simulink model "rev0BB"  (R2017b)
settings: Solver=FixedStepDiscrete  StartTime=0  StopTime=(((preLen+100+dataLenSymbols)*1+pad_first*3)*basePer)  RelTol=1e-3
values from neighbouring files (symbols this model uses):
  ack_stf_len_symbols = length(x_ACK_STF)    [rev0BB_setup.m]
  agc_delay_lag = 32    [rev0BB_setup.m]
  agc_detector_coef = ones(1,agc_detector_taps)./agc_detector_taps    [rev0BB_setup.m]
  agc_on = true    [rev0BB_startup.m]
  agc_sat_low = -agcSaturation    (= -12)    [rev0BB_setup.m]
  agc_sat_up = agcSaturation    (= 12)    [rev0BB_setup.m]
  agcDesired = 0    [rev0BB_setup.m]
  agcExpDomain = agcSaturation    (= 12)    [rev0BB_setup.m]
  agcExpResolution = 2^-5    (= 0.03125)    [rev0BB_setup.m]
  agcPwrAvgNum = 128    [rev0BB_setup.m]
  agcSaturation = 12    [rev0BB_setup.m]
  agcSettleThresh = 0.65    [rev0BB_setup.m]
  agcStep = 2^-8    (= 0.00390625)    [rev0BB_setup.m]
  atanDomain = 5    [rev0BB_setup.m]
  atanDomainTiming = 256    [rev0BB_setup.m]
  atanResolution = 2^-9    (= 0.001953125)    [rev0BB_setup.m]
  atanResolutionTiming = 2^-5    (= 0.03125)    [rev0BB_setup.m]
  averaging_num = ones(1, averaging_samples)    [rev0BB_setup.m]
  averaging_samples = 128    [rev0BB_setup.m]
  awgnSeed = abs(dBSnrRange(dBSnrInd)*1000+trial+10000000)    [plotBer.m]    (also in rev0BB_startup.m = 67)
  basePer = 1/baseFreq    (= 5e-08)    [rev0BB_setup.m]
  bitsPerSymbolHeader = log2(radixHeader)    [rev0BB_setup.m]
  bitsPerSymbolMax = log2(radixMax)    [rev0BB_setup.m]
  cal_sig_i_mult = 1.0    (= 1)    [rev0BB_startup.m]
  cal_sig_i_offset = 0.0    (= 0)    [rev0BB_startup.m]
  cal_sig_q_mult = 1.0    (= 1)    [rev0BB_startup.m]
  cal_sig_q_offset = 0.0    (= 0)    [rev0BB_startup.m]
  cefEarlyWarning = 256    [rev0BB_setup.m]
  cefLen = length(x_CEF)    [rev0BB_setup.m]
  channelFIR = zeros(1, round(maxSampleDelay)+1)    [rev0BB_startup.m]
  coarseCFOAdaptDelay = 1    [rev0BB_setup.m]
  cr_i = 0.020    (= 0.02)    [rev0BB_setup.m]
  cr_i_preamp = 2^-9    (= 0.001953125)    [rev0BB_setup.m]
  cr_int1_sat_low = -cr_integrator1_saturation    (= -0.6)    [rev0BB_setup.m]
  cr_int1_sat_up = cr_integrator1_saturation    (= 0.6)    [rev0BB_setup.m]
  cr_integrator1_decay = 1    [rev0BB_setup.m]
  cr_integrator1_saturation = 0.6    [rev0BB_setup.m]
  cr_mult_pipeline = 0    [rev0BB_setup.m]
  cr_p = 0.015    [rev0BB_setup.m]
  cr_sat2_low = -cr_saturation2    (= -0.6)    [rev0BB_setup.m]
  cr_sat2_up = cr_saturation2    (= 0.6)    [rev0BB_setup.m]
  cr_smooth_num = (1/cr_smooth_samples).*ones(1, cr_smooth_samples)    [rev0BB_setup.m]
  D_128 = [ 1,  8,  2,  4, 16, 32, 64]    [golay.m]    (also in rev0BB_setup.m)
  D_32 = [ 1,  4,  8,  2, 16]    [golay.m]    (also in rev0BB_setup.m)
  dataLenSymbols = header_len_bytes*8/bitsPerSymbolHeader + frame_len_bytes*8/bitsPerSymbol    [rev0BB_setup.m]
  default_channel = 3    [rev0BB_setup.m]
  dmm_coefs = ones(1,dmm_samples)./dmm_samples    [rev0BB_setup.m]
  dst_field_len = 8    [rev0BB_setup.m]
  expDomain = 3.3    [rev0BB_setup.m]
  expResolution = 2^-5    (= 0.03125)    [rev0BB_setup.m]
  expTol = .1    (= 0.1)    [rev0BB_setup.m]
  flush_delay = regular_pipeline*2+mult_pipeline+4    (= 4)    [rev0BB_setup.m]
  frac_lut_domain = 256    [rev0BB_setup.m]
  frac_lut_domain_cr = 64    [rev0BB_setup.m]
  frac_lut_range_max = 512    [rev0BB_setup.m]
  frac_lut_range_max_coarse_cfo = 127    [rev0BB_setup.m]
  frac_lut_range_max_cr = 127    [rev0BB_setup.m]
  frac_lut_range_min = -frac_lut_range_max    (= -512)    [rev0BB_setup.m]
  frac_lut_range_min_coarse_cfo = -frac_lut_range_max_coarse_cfo    (= -127)    [rev0BB_setup.m]
  frac_lut_range_min_cr = -frac_lut_range_max_cr    (= -127)    [rev0BB_setup.m]
  frac_lut_table_breaks = -frac_lut_domain:frac_lut_res:(frac_lut_domain-1)    [rev0BB_setup.m]
  frac_lut_table_breaks_coarse_cfo = -frac_lut_domain_coarse_cfo:frac_lut_res_coarse_cfo:(frac_lut_domain_coarse_cfo-1)    [rev0BB_setup.m]
  frac_lut_table_breaks_cr = -frac_lut_domain_cr:frac_lut_res_cr:(frac_lut_domain_cr-1)    [rev0BB_setup.m]
  frac_lut_table_data = 1./frac_lut_table_breaks    [rev0BB_setup.m]
  frac_lut_table_data_coarse_cfo = 1./frac_lut_table_breaks_coarse_cfo    [rev0BB_setup.m]
  frac_lut_table_data_cr = 1./frac_lut_table_breaks_cr    [rev0BB_setup.m]
  freeze_en_agc = true    [rev0BB_startup.m]
  freeze_en_cr_int1 = false    [rev0BB_startup.m]
  freeze_en_cr_int2 = false    [rev0BB_startup.m]
  freeze_en_cr_phase = false    [rev0BB_startup.m]
  freeze_en_tr_int1 = false    [rev0BB_startup.m]
  freeze_en_tr_int2 = false    [rev0BB_startup.m]
  freeze_en_tr_phase = false    [rev0BB_startup.m]
  freeze_on_cef_done = true    [rev0BB_startup.m]
  freeze_on_stf_done = false    [rev0BB_startup.m]
  freeze_on_valid = true    [rev0BB_startup.m]
  golay_type = 32    [rev0BB_setup.m]
  guardInt = int16(4)    [rev0BB_setup.m]
  guardTol = int16(5)    [rev0BB_setup.m]
  header_len_bytes = 8    [rev0BB_setup.m]
  lineWidth = 60    [rev0BB_setup.m]
  lmsEqDepth = 38    [rev0BB_setup.m]
  lmsStep_init = 0.006    [rev0BB_setup.m]
  lmsStep_meta = (lmsStep_final - lmsStep_init)/cefLen    [rev0BB_setup.m]
  lnDomain = 16    [rev0BB_setup.m]
  lnResolution = 2^-5    (= 0.03125)    [rev0BB_setup.m]
  local_node_id = 2    [rev0BB_startup.m]
  maxMsgSize = length(xSpectrum_PRE)+dataLenSymbols+300    [rev0BB_setup.m]
  minSTFPeaks = 3    [rev0BB_setup.m]
  mod_scheme_len_bytes = 1    [rev0BB_setup.m]
  modBPS = [1, 2, 4]    [rev0BB_setup.m]
  modKeys = [0, 1, 2]    [rev0BB_setup.m]
  mult_pipeline = 0    [rev0BB_setup.m]
  overSampleFreq = 80e6    (= 80000000)    [rev0BB_setup.m]
  overSamplePer = 1/overSampleFreq    (= 1.25e-08)    [rev0BB_setup.m]
  pad_first = 1000    [createTestVectors.m]
  post_cr_i_offset = 0    [rev0BB_startup.m]
  post_cr_q_offset = 0    [rev0BB_startup.m]
  preambleSequentialDetect = 2    [rev0BB_setup.m]
  preLen = length(x_PRE)    [rev0BB_setup.m]
  qam16_demod_scale_factor = qam16_hdl_distance/qam16_power_normalized_distance    [rev0BB_setup.m]
  rcRxFilt = [0.000303163120401141 -0.00118915940834234 -0.00187387637177 -0.00124167532697737 0.00029186889076529 0.00164526160586517 0.00182432050803312 0.000652133621739543 -0.00105668254004908 -0.00204011570659167 -0.00150058088768918 0.00026138356356816 0.0019831869994874 0.00231075800085521 0.000821993419120097 -0.00154687337975486 -0.00305430783933469 -0.00238186490079127 0.000301216962040692 0.00325307 ...(+2001 chars)    [rev0BB_setup.m]
  rcTxFilt = [0.000303163120401141 -0.00118915940834234 -0.00187387637177 -0.00124167532697737 0.00029186889076529 0.00164526160586517 0.00182432050803312 0.000652133621739543 -0.00105668254004908 -0.00204011570659167 -0.00150058088768918 0.00026138356356816 0.0019831869994874 0.00231075800085521 0.000821993419120097 -0.00154687337975486 -0.00305430783933469 -0.00238186490079127 0.000301216962040692 0.00325307 ...(+2001 chars)    [rev0BB_setup.m]
  regular_pipeline = 0    [rev0BB_setup.m]
  rx_gain = 1    [rev0BB_setup.m]
  rx_gain_i = 1    [rev0BB_setup.m]
  rx_gain_q = 1    [rev0BB_setup.m]
  rx_impare_i_offset = 0    [rev0BB_startup.m]
  rx_impare_i_scale = 1    [rev0BB_startup.m]
  rx_impare_q_offset = 0    [rev0BB_startup.m]
  rx_impare_q_scale = 1    [rev0BB_startup.m]
  rx_offset_correction_i = 0    [rev0BB_startup.m]
  rx_offset_correction_q = 0    [rev0BB_startup.m]
  sin_source_amp = 1    [rev0BB_setup.m]
  sin_source_freq = 250e6/16    (= 15625000)    [rev0BB_setup.m]
  slowPer = overSamplePer*slowSample    (= 2.5e-08)    [rev0BB_setup.m]
  std_pkt_type = 0    [rev0BB_setup.m]
  stfLen = length(x_STF)    [rev0BB_setup.m]
  testMsg = cat(1, xCTRL_PRE_adj, header, payload)    [plotBer.m]
  timing_i = 0.25    [rev0BB_setup.m]
  ... (+25 more)
undefined symbols (not defined in the file or in its folder): cr_integrator2_saturation, doppler, i, magnitude, useFadingChannel
libraries: helperLib x128, simulink x90, golayLib x34, dspsigops x32, commfilt2 x27, commdigbbndpm3 x8, hdlsllib x6, dsparch4 x4, commdigbbndam3 x4, commchan3 x2, commrflib2 x2, commcrc2 x2
(part 10 of 10)

== stateflow chart rev0BB/receiver/rx_select/rx_select ==
  settings: executeAtInitialization=1
  state Rx1
    entry:
    select = uint8(0);
    receiving = true;
    count = count + uint32(1);
  state Idle
    entry:
    select = uint8(default_channel);
    receiving = false;
    err = false;
    count = uint32(0);
  state Err
    entry:
    err = true;
  state Rx2
    entry:
    select = uint8(1);
    receiving = true;
    count = count + uint32(1);
  state Rx3
    entry:
    select = uint8(2);
    receiving = true;
    count = count + uint32(1);
  Rx3 -> Idle [order 1] : [done == true]
  Rx2 -> Idle [order 1] : [done == true]
  Rx1 -> Idle [order 1] : [done == true]
  Idle -> Rx1 [order 1] : [preamble_detect1 == true]
  (default) -> Idle
  Idle -> Rx2 [order 2] : [preamble_detect2 == true]
  Rx1 -> Err [order 2] : [count > maxMsgSize*4]
  Idle -> Rx3 [order 3] : [preamble_detect3 == true]
  Rx1 -> Rx1 [order 3]
  Err -> Idle
  Rx2 -> Err [order 2] : [count > maxMsgSize*4]
  Rx3 -> Err [order 2] : [count > maxMsgSize*4]
  Rx2 -> Rx2 [order 3]
  Rx3 -> Rx3 [order 3]
  data: default_channel parameter; maxMsgSize parameter; preamble_detect3 input; preamble_detect2 input; preamble_detect1 input; receiving output; select output uint8; err output; count local; done input

== stateflow chart rev0BB/receiver/slow_rx_baseband_outer/slow_rx_baseband_enabled/slow_rx_baseband/header_parse_ack_decision/header_parse ==
  settings: executeAtInitialization=1
  state ParseLen
    entry:
    len = bitor(bitsrl(len, bitsPerSymbolHeader), bitsll(uint16(data), 16-bitsPerSymbolHeader));
    counter = counter + uint8(bitsPerSymbolHeader);
  state Hold
    entry:
    payload = true;
    payload_early=true;
    done_parsing = true;
  state ParseNet_Id
    entry:
    net_id = bitor(bitsrl(len, bitsPerSymbolHeader), bitsll(uint16(data), 16-bitsPerSymbolHeader));
    counter = counter + uint8(bitsPerSymbolHeader);
  state ParseDst
    entry:
    dst = bitor(bitsrl(dst, bitsPerSymbolHeader), bitsll(data, 8-bitsPerSymbolHeader));
    counter = counter + uint8(bitsPerSymbolHeader);
  state ParseSrc
    entry:
    src = bitor(bitsrl(src, bitsPerSymbolHeader), bitsll(data, 8-bitsPerSymbolHeader));
    counter = counter + uint8(bitsPerSymbolHeader);
  state ParseModType
    entry:
    mod_type = bitor(bitsrl(mod_type, bitsPerSymbolHeader),bitsll(data, 8-bitsPerSymbolHeader));
    counter = counter + uint8(bitsPerSymbolHeader);
  state Waiting
    entry:
    counter = uint8(0);
    mod_type = uint8(0);
    mod_type_valid = false;
    type = uint8(0);
    type_valid = false;
    src = uint8(0);
    src_valid = false;
    dst = uint8(0);
    dst_valid = false;
    net_id = uint16(0);
    net_id_valid = false;
    len = uint16(0);
    len_valid = false;
    done_parsing = false;
    payload = false;
    payload_early=false;
  state ParseType
    entry:
    type = bitor(bitsrl(type, bitsPerSymbolHeader),bitsll(data, 8-bitsPerSymbolHeader));
    counter = counter + uint8(bitsPerSymbolHeader);
  state ParseLenLast
    entry:
    len = bitor(bitsrl(len, bitsPerSymbolHeader), bitsll(uint16(data), 16-bitsPerSymbolHeader));
    len_valid = true;
    payload_early=true;
    counter = uint8(0);
  state ParseModTypeLast
    entry:
    mod_type = bitor(bitsrl(mod_type, bitsPerSymbolHeader), bitsll(data, 8-bitsPerSymbolHeader));
    mod_type_valid = true;
    counter = uint8(0);
  state ParseTypeLast
    entry:
    type = bitor(bitsrl(type, bitsPerSymbolHeader), bitsll(data, 8-bitsPerSymbolHeader));
    type_valid = true;
    counter = uint8(0);
  state ParseNet_IdLast
    entry:
    net_id = bitor(bitsrl(len, bitsPerSymbolHeader), bitsll(uint16(data), 16-bitsPerSymbolHeader));
    net_id_valid = true;
    counter = uint8(0);
  state ParseSrcLast
    entry:
    src = bitor(bitsrl(src, bitsPerSymbolHeader), bitsll(data, 8-bitsPerSymbolHeader));
    src_valid = true;
    counter = uint8(0);
  state ParseDstLast
    entry:
    dst = bitor(bitsrl(dst, bitsPerSymbolHeader), bitsll(data, 8-bitsPerSymbolHeader));
    dst_valid = true;
    counter = uint8(0);
  ParseLenLast -> Waiting [order 1] : [rst==true]
  ParseNet_IdLast -> Waiting [order 1] : [rst==true]
  ParseNet_Id -> Waiting [order 1] : [rst==true]
  ParseLen -> Waiting [order 1] : [rst==true]
  ParseDstLast -> Waiting [order 1] : [rst==true]
  ParseDst -> Waiting [order 1] : [rst==true]
  ParseSrcLast -> Waiting [order 1] : [rst==true]
  ParseSrc -> Waiting [order 1] : [rst==true]
  ParseTypeLast -> Waiting [order 1] : [rst==true]
  ParseType -> Waiting [order 1] : [rst==true]
  ParseModTypeLast -> Waiting [order 1] : [rst==true]
  ParseLen -> ParseLen [order 3] : [counter < 16-bitsPerSymbolHeader ]
  Hold -> Hold [order 2]
  ParseNet_Id -> ParseNet_Id [order 3] : [counter < 16-bitsPerSymbolHeader ]
  ParseModType -> Waiting [order 2] : [rst==true]
  ParseDst -> ParseDst [order 3] : [counter < 8-bitsPerSymbolHeader ]
  ParseSrc -> ParseSrc [order 3] : [counter < 8-bitsPerSymbolHeader ]
  ParseModType -> ParseModType [order 3] : [counter < 8-bitsPerSymbolHeader ]
  ParseType -> ParseType [order 3] : [counter < 8-bitsPerSymbolHeader ]
  (default) -> Waiting
  ParseNet_IdLast -> ParseLen [order 2]
  ParseLen -> ParseLenLast [order 2] : [counter >= 16-bitsPerSymbolHeader ]
  ParseLenLast -> Hold [order 2]
  ParseDstLast -> ParseNet_Id [order 2]
  ParseNet_Id -> ParseNet_IdLast [order 2] : [counter >= 16-bitsPerSymbolHeader ]
  Waiting -> ParseModType [order 1] : [valid==true]
  Hold -> Waiting [order 1] : [rst == true]
  ParseModTypeLast -> ParseType [order 2]
  ParseType -> ParseTypeLast [order 2] : [counter >= 8-bitsPerSymbolHeader ]
  ParseModType -> ParseModTypeLast [order 1] : [counter >= 8-bitsPerSymbolHeader ]
  ParseTypeLast -> ParseSrc [order 2]
  ParseSrc -> ParseSrcLast [order 2] : [counter >= 8-bitsPerSymbolHeader ]
  ParseSrcLast -> ParseDst [order 2]
  ParseDst -> ParseDstLast [order 2] : [counter >= 8-bitsPerSymbolHeader ]
  Waiting -> Waiting [order 2] : [valid==false]
  data: mod_type_valid output boolean; data input uint8; valid input boolean; type_valid output boolean; src_valid output boolean; dst_valid output boolean; len_valid output boolean; done_parsing output boolean; mod_type output uint8; counter local; type output uint8; src output uint8; dst output uint8; len output uint16; rst input boolean; bitsPerSymbolHeader parameter int8; payload output boolean; payload_early output boolean; net_id_valid output boolean; net_id output uint16

== stateflow chart rev0BB/ack_generator/ack_generator ==
  settings: executeAtInitialization=1
  state GaLast
    entry:
    dst_counter = dst_counter + uint8(1);
    dst_internal = bitsrl(dst_internal, 1);
    data_out = GaGen(counter+1);
    counter = uint16(0);
    valid_out = true;
    tail=false;
    last = false;
  state Ga
    entry:
    data_out = GaGen(counter+1);
    counter = counter + uint16(1);
    valid_out = true;
    tail=false;
    last = false;
  state STF
    entry:
    data_out = stfGen(counter+1);
    counter = counter + uint16(1);
    valid_out = true;
    tail=false;
    last = false;
  state STFLast
    entry:
    data_out = stfGen(counter+1);
    counter = uint16(0);
    valid_out = true;
    tail=false;
    last = false;
  state Tail
    entry:
    data_out = int32(0);
    counter = counter + uint16(1);
    tail=true;
    valid_out = true;
    last = false;
  state TailLast
    entry:
    data_out = int32(0);
    counter = uint16(0);
    tail=true;
    valid_out = true;
    last = true;
  state Waiting
    entry:
    dst_internal = uint8(0);
    valid_out = false;
    data_out = int32(0);
    counter = uint16(0);
    dst_counter = uint8(0);
    tx_chan = uint8(default_channel);
    tail=false;
    last = false;
  state Triggered
    entry:
    dst_internal = dst_in;
    valid_out = false;
    data_out = int32(0);
    tail=false;
    last = false;
    tx_chan = ack_chan;
  state Gb
    entry:
    data_out = GbGen(counter+1);
    counter = counter + uint16(1);
    valid_out = true;
    tail=false;
    last = false;
  state GbLast
    entry:
    dst_counter = dst_counter + uint8(1);
    dst_internal = bitsrl(dst_internal, 1);
    data_out = GbGen(counter+1);
    counter = uint16(0);
    valid_out = true;
    tail=false;
    last = false;
  TailLast -> Waiting
  Tail -> Waiting [order 1] : [cancel==true]
  GaLast -> Waiting [order 1] : [cancel==true]
  Ga -> Ga [order 3] : [counter < ack_stf_len_symbols-1]
  Ga -> Waiting [order 1] : [cancel==true]
  STFLast -> Waiting [order 3] : [cancel==true]
  STFLast -> Ga [order 1] : [mod(dst_internal,2)==0]
  Ga -> GaLast [order 2] : [counter >= golay_type-1]
  GaLast -> Tail [order 4] : [dst_counter >= dst_field_len]
  STF -> Waiting [order 1] : [cancel==true]
  GbLast -> Ga [order 2] : [dst_counter < dst_field_len && mod(dst_internal,2)==0 ]
  GaLast -> Ga [order 3] : [dst_counter < dst_field_len && mod(dst_internal,2)==0 ]
  GaLast -> Gb [order 2] : [dst_counter < dst_field_len && mod(dst_internal,2)==1 ]
  Triggered -> Waiting [order 1] : [cancel==true]
  (default) -> Waiting
  Triggered -> STF [order 2]
  Waiting -> Triggered : [ack==true]
  STF -> STFLast [order 3] : [counter >= ack_stf_len_symbols-1]
  Tail -> TailLast [order 3] : [counter >= flush_delay-1]
  STFLast -> Gb [order 2] : [mod(dst_internal,2)==1]
  GbLast -> Waiting [order 1] : [cancel==true]
  Gb -> Waiting [order 1] : [cancel==true]
  STF -> STF [order 2] : [counter < ack_stf_len_symbols-1]
  GbLast -> Tail [order 4] : [dst_counter >= dst_field_len]
  Tail -> Tail [order 2] : [counter < flush_delay-1]
  GbLast -> Gb [order 3] : [dst_counter < dst_field_len && mod(dst_internal,2)==1 ]
  Gb -> GbLast [order 2] : [counter >= golay_type-1]
  Gb -> Gb [order 3] : [counter < ack_stf_len_symbols-1]
  data: ind function_input; symb function_output boolean; ind function_input; symb function_output boolean; ind function_input; symb function_output boolean; ack input boolean; cancel input boolean; dst_field_len parameter; ack_stf_len_symbols parameter; data_out output int32; valid_out output boolean; counter local uint16; dst_internal local uint8; dst_counter local uint8; flush_delay parameter; tail output boolean; last output boolean; dst_in input uint8; golay_type parameter; ack_chan input uint8; tx_chan output uint8; default_channel parameter
  function symb = stfGen(ind):
    | function symb = stfGen(ind)
    | %128
    | % Ga_128 = [+1, +1, -1, -1, -1, -1, -1, -1, -1, +1, -1, +1, +1, -1, -1, +1, +1, +1, -1, -1, +1, +1, +1, +1, -1, +1, -1, +1, -1, +1, +1, -1, -1, -1, +1, +1, +1, +1, +1, +1, +1, -1, +1, -1, -1, +1, +1, -1, +1, +1, -1, -1, +1, +1, +1, +1, -1, +1, -1, +1, -1, +1, +1, -1, +1, +1, -1, -1, -1, -1, -1, -1, -1, +1, -1, +1, +1, -1, -1, +1, +1, +1, -1, -1, +1, +1, +1, +1, -1, +1, -1, +1, -1, +1, +1, -1, +1, +1, -1, -1, -1, -1, -1, -1, -1, +1, -1, +1, +1, -1, -1, +1, -1, -1, +1, +1, -1, -1, -1, -1, +1, -1, +1, -1, +1, -1, -1, +1];
    | % Gb_128 = [-1, -1, +1, +1, +1, +1, +1, +1, +1, -1, +1, -1, -1, +1, +1, -1, -1, -1, +1, +1, -1, -1, -1, -1, +1, -1, +1, -1, +1, -1, -1, +1, +1, +1, -1, -1, -1, -1, -1, -1, -1, +1, -1, +1, +1, -1, -1, +1, -1, -1, +1, +1, -1, -1, -1, -1, +1, -1, +1, -1, +1, -1, -1, +1, +1, +1, -1, -1, -1, -1, -1, -1, -1, +1, -1, +1, +1, -1, -1, +1, +1, +1, -1, -1, +1, +1, +1, +1, -1, +1, -1, +1, -1, +1, +1, -1, +1, +1, -1, -1, -1, -1, -1, -1, -1, +1, -1, +1, +1, -1, -1, +1, -1, -1, +1, +1, -1, -1, -1, -1, +1, -1, +1, -1, +1, -1, -1, +1];
    | % 
    | % Gu_512 = cat(2, -Gb_128, -Ga_128, Gb_128, -Ga_128);
    | % Gv_512 = cat(2, -Gb_128, Ga_128, -Gb_128, -Ga_128);
    | % Gv_128 = Gv_512(1:1:128);
    | 
    | % xSpectrum_CEF = cat(2, Gu_512, Gv_512, Gu_512, Gv_512, Gu_512, Gv_512, Gu_512, Gv_512, Gu_512, Gv_512, Gv_128);
    | % xSpectrum_CEF = cat(2, Gu_512, Gv_512, Gv_512);
    | 
    | %32
    | Ga_32  = [+1, +1, +1, +1, +1, -1, +1, -1, -1, -1, +1, +1, +1, -1, -1, +1, +1, +1, -1, -1, +1, -1, -1, +1, -1, -1, -1, -1, +1, -1, +1, -1];
    | Gb_32  = [-1, -1, -1, -1, -1, +1, -1, +1, +1, +1, -1, -1, -1, +1, +1, -1, +1, +1, -1, -1, +1, -1, -1, +1, -1, -1, -1, -1, +1, -1, +1, -1];
    | 
    | Gu_128_s = cat(2, -Gb_32, -Ga_32, Gb_32, -Ga_32);
    | Gv_128_s = cat(2, -Gb_32, Ga_32, -Gb_32, -Ga_32);
    | 
    | nSpectrumAck_STFRepCount_short = 13;
    | nSpectrumAck_STFRep_short = 0:1:(nSpectrumAck_STFRepCount_short*32-1);
    | nSpectrumAck_STFNeg_short = (nSpectrumAck_STFRepCount_short*32):1:((nSpectrumAck_STFRepCount_short+1)*32-1);
    | nSpectrumAck_STFFin_short = ((nSpectrumAck_STFRepCount_short+1)*32):1:((nSpectrumAck_STFRepCount_short+2)*32-1);
    | 
    | xSpectrumAck_STF_short = cat(2, Gb_32(mod(nSpectrumAck_STFRep_short, 32)+1), -Gb_32(mod(nSpectrumAck_STFNeg_short, 32)+1), -Ga_32(mod(nSpectrumAck_STFFin_short, 32)+1)); %+1 is for matlab
    | xSpectrumAck_STF_short = cat(2, xSpectrumAck_STF_short, Ga_32);
    | 
    | xSpectrumAck_STF_short = (xSpectrumAck_STF_short-1)./(-2);
    | 
    | symb = int32(xSpectrumAck_STF_short(ind));
    | 
    | end
  function symb = GaGen(ind):
    | function symb = GaGen(ind)
    | %128
    | % Ga_128 = [+1, +1, -1, -1, -1, -1, -1, -1, -1, +1, -1, +1, +1, -1, -1, +1, +1, +1, -1, -1, +1, +1, +1, +1, -1, +1, -1, +1, -1, +1, +1, -1, -1, -1, +1, +1, +1, +1, +1, +1, +1, -1, +1, -1, -1, +1, +1, -1, +1, +1, -1, -1, +1, +1, +1, +1, -1, +1, -1, +1, -1, +1, +1, -1, +1, +1, -1, -1, -1, -1, -1, -1, -1, +1, -1, +1, +1, -1, -1, +1, +1, +1, -1, -1, +1, +1, +1, +1, -1, +1, -1, +1, -1, +1, +1, -1, +1, +1, -1, -1, -1, -1, -1, -1, -1, +1, -1, +1, +1, -1, -1, +1, -1, -1, +1, +1, -1, -1, -1, -1, +1, -1, +1, -1, +1, -1, -1, +1];
    | % Gb_128 = [-1, -1, +1, +1, +1, +1, +1, +1, +1, -1, +1, -1, -1, +1, +1, -1, -1, -1, +1, +1, -1, -1, -1, -1, +1, -1, +1, -1, +1, -1, -1, +1, +1, +1, -1, -1, -1, -1, -1, -1, -1, +1, -1, +1, +1, -1, -1, +1, -1, -1, +1, +1, -1, -1, -1, -1, +1, -1, +1, -1, +1, -1, -1, +1, +1, +1, -1, -1, -1, -1, -1, -1, -1, +1, -1, +1, +1, -1, -1, +1, +1, +1, -1, -1, +1, +1, +1, +1, -1, +1, -1, +1, -1, +1, +1, -1, +1, +1, -1, -1, -1, -1, -1, -1, -1, +1, -1, +1, +1, -1, -1, +1, -1, -1, +1, +1, -1, -1, -1, -1, +1, -1, +1, -1, +1, -1, -1, +1];
    | % 
    | % Gu_512 = cat(2, -Gb_128, -Ga_128, Gb_128, -Ga_128);
    | % Gv_512 = cat(2, -Gb_128, Ga_128, -Gb_128, -Ga_128);
    | % Gv_128 = Gv_512(1:1:128);
    | 
    | % xSpectrum_CEF = cat(2, Gu_512, Gv_512, Gu_512, Gv_512, Gu_512, Gv_512, Gu_512, Gv_512, Gu_512, Gv_512, Gv_128);
    | % xSpectrum_CEF = cat(2, Gu_512, Gv_512, Gv_512);
    | 
    | %32
    | Ga_32  = ([+1, +1, +1, +1, +1, -1, +1, -1, -1, -1, +1, +1, +1, -1, -1, +1, +1, +1, -1, -1, +1, -1, -1, +1, -1, -1, -1, -1, +1, -1, +1, -1]-1)./(-2);
    | 
    | symb = int32(Ga_32(ind));
    | 
    | end
  function symb = GbGen(ind):
    | function symb = GbGen(ind)
    | %128
    | % Ga_128 = [+1, +1, -1, -1, -1, -1, -1, -1, -1, +1, -1, +1, +1, -1, -1, +1, +1, +1, -1, -1, +1, +1, +1, +1, -1, +1, -1, +1, -1, +1, +1, -1, -1, -1, +1, +1, +1, +1, +1, +1, +1, -1, +1, -1, -1, +1, +1, -1, +1, +1, -1, -1, +1, +1, +1, +1, -1, +1, -1, +1, -1, +1, +1, -1, +1, +1, -1, -1, -1, -1, -1, -1, -1, +1, -1, +1, +1, -1, -1, +1, +1, +1, -1, -1, +1, +1, +1, +1, -1, +1, -1, +1, -1, +1, +1, -1, +1, +1, -1, -1, -1, -1, -1, -1, -1, +1, -1, +1, +1, -1, -1, +1, -1, -1, +1, +1, -1, -1, -1, -1, +1, -1, +1, -1, +1, -1, -1, +1];
    | % Gb_128 = [-1, -1, +1, +1, +1, +1, +1, +1, +1, -1, +1, -1, -1, +1, +1, -1, -1, -1, +1, +1, -1, -1, -1, -1, +1, -1, +1, -1, +1, -1, -1, +1, +1, +1, -1, -1, -1, -1, -1, -1, -1, +1, -1, +1, +1, -1, -1, +1, -1, -1, +1, +1, -1, -1, -1, -1, +1, -1, +1, -1, +1, -1, -1, +1, +1, +1, -1, -1, -1, -1, -1, -1, -1, +1, -1, +1, +1, -1, -1, +1, +1, +1, -1, -1, +1, +1, +1, +1, -1, +1, -1, +1, -1, +1, +1, -1, +1, +1, -1, -1, -1, -1, -1, -1, -1, +1, -1, +1, +1, -1, -1, +1, -1, -1, +1, +1, -1, -1, -1, -1, +1, -1, +1, -1, +1, -1, -1, +1];
    | % 
    | % Gu_512 = cat(2, -Gb_128, -Ga_128, Gb_128, -Ga_128);
    | % Gv_512 = cat(2, -Gb_128, Ga_128, -Gb_128, -Ga_128);
    | % Gv_128 = Gv_512(1:1:128);
    | 
    | % xSpectrum_CEF = cat(2, Gu_512, Gv_512, Gu_512, Gv_512, Gu_512, Gv_512, Gu_512, Gv_512, Gu_512, Gv_512, Gv_128);
    | % xSpectrum_CEF = cat(2, Gu_512, Gv_512, Gv_512);
    | 
    | %32
    | Gb_32  = ([-1, -1, -1, -1, -1, +1, -1, +1, +1, +1, -1, -1, -1, +1, +1, -1, +1, +1, -1, -1, +1, -1, -1, +1, -1, -1, -1, -1, +1, -1, +1, -1]-1)./(-2);
    | 
    | symb = int32(Gb_32(ind));
    | 
    | end

== stateflow chart rev0BB/receiver/slow_rx_baseband_outer/slow_rx_baseband_enabled/slow_rx_baseband/mod_data_buffer/header_parse ==
  settings: executeAtInitialization=1
  state Exe
    note: Used if Max Modulation Scheme is BPSK
    note: Note: It is assumed that the header will exactly fit into the packed representation with no padding required. This simplifies this decoder.
    state HeaderPassThrough
      entry:
      packed_data = data;
      counter = uint8(0);
      valid = true;
      decoding=true;
    state PayloadPassThrough
      entry:
      packed_data = data;
      counter = uint8(0);
      valid = true;
    state PayloadPassThroughLast
      entry:
      packed_data = data;
      counter = uint8(0);
      valid = true;
      last_out=true;
    state FillHeaderOutput
      entry:
      packed_data = bitor(bitsrl(packed_data, bitsPerSymbolHeader),bitsll(data, bitsPerSymbolMax-bitsPerSymbolHeader));
      counter = counter + uint8(bitsPerSymbolHeader);
      valid = true;
      decoding=true;
    state FillPayloadOutput
      entry:
      packed_data = bitor(bitsrl(packed_data, bitsPerSymbolMod),bitsll(data, bitsPerSymbolMax-bitsPerSymbolMod));
      counter = counter + uint8(bitsPerSymbolMod);
      valid = true;
    state FillHeaderFirst
      entry:
      packed_data = bitsll(data, bitsPerSymbolMax-bitsPerSymbolHeader);
      counter = uint8(bitsPerSymbolHeader);
      valid = false;
    state FillHeaderMid
      entry:
      packed_data = bitor(bitsrl(packed_data, bitsPerSymbolHeader),bitsll(data, bitsPerSymbolMax-bitsPerSymbolHeader));
      counter = counter + uint8(bitsPerSymbolHeader);
      valid = false;
    state FillPayloadFirst
      entry:
      packed_data = bitsll(data, bitsPerSymbolMax-bitsPerSymbolMod);
      counter = uint8(bitsPerSymbolMod);
      valid = false;
    state FillPayloadMid
      entry:
      packed_data = bitor(bitsrl(packed_data, bitsPerSymbolMod),bitsll(data, bitsPerSymbolMax-bitsPerSymbolMod));
      counter = counter + uint8(bitsPerSymbolMod);
      valid = false;
    state FillPayloadOutputLast
      entry:
      packed_data = bitor(bitsrl(packed_data, bitsPerSymbolMod),bitsll(data, bitsPerSymbolMax-bitsPerSymbolMod));
      counter = counter + uint8(bitsPerSymbolMod);
      valid = true;
      last_out = true;
    state Err
      entry:
      last_out=true;
      err = true;
    HeaderPassThrough -> HeaderPassThrough [order 3]
    PayloadPassThrough -> PayloadPassThrough [order 2]
    HeaderPassThrough -> PayloadPassThrough [order 1] : [payload == true && bitsPerSymbolMod == bitsPerSymbolMax]
    PayloadPassThrough -> PayloadPassThroughLast [order 1] : [last_in==true]
    FillHeaderOutput -> PayloadPassThrough [order 2] : [payload == true && bitsPerSymbolMod == bitsPerSymbolMax]
    HeaderPassThrough -> FillPayloadFirst [order 2] : [payload == true && bitsPerSymbolMod ~= bitsPerSymbolMax]
    FillHeaderMid -> FillHeaderMid [order 2]
    FillPayloadMid -> FillPayloadMid [order 4]
    FillHeaderFirst -> FillHeaderMid [order 2]
    FillPayloadFirst -> FillPayloadMid [order 3]
    FillHeaderMid -> FillHeaderOutput [order 1] : [counter >=bitsPerSymbolMax-bitsPerSymbolHeader ]
    FillHeaderOutput -> FillPayloadFirst [order 1] : [payload == true && bitsPerSymbolMod ~= bitsPerSymbolMax]
    FillPayloadMid -> FillPayloadOutput [order 1] : [counter >=bitsPerSymbolMax-bitsPerSymbolMod && last_in ==false ]
    FillPayloadMid -> FillPayloadOutputLast [order 2] : [counter >=bitsPerSymbolMax-bitsPerSymbolMod && last_in ==true ]
    FillPayloadOutput -> Err [order 1] : [last_in ==true]
    FillHeaderOutput -> FillHeaderFirst [order 3]
    FillHeaderFirst -> FillHeaderOutput [order 1] : [counter >=bitsPerSymbolMax-bitsPerSymbolHeader ]
    FillPayloadFirst -> FillPayloadOutputLast [order 2] : [last_in ==true]
    FillPayloadOutput -> FillPayloadFirst [order 2]
    FillPayloadFirst -> FillPayloadOutput [order 1] : [counter >=bitsPerSymbolMax-bitsPerSymbolMod && last_in ==false ]
    FillPayloadMid -> Err [order 3] : [counter < bitsPerSymbolMax-bitsPerSymbolMod && last_in ==true ]
  state Waiting
    entry:
    counter = uint8(0);
    packed_data = uint8(0);
    valid = false;
    last_out=false;
    decoding=false;
    err=false;
  PayloadPassThroughLast -> Waiting
  Exe -> Waiting : [rst == true]
  Waiting -> HeaderPassThrough [order 2] : [header==true && bitsPerSymbolMax == 1]
  (default) -> Waiting
  Waiting -> FillHeaderFirst [order 1] : [header==true && bitsPerSymbolMax ~= 1]
  Err -> Waiting
  FillPayloadOutputLast -> Waiting
  data: last_in input boolean; header input boolean; bitsPerSymbolMax parameter uint8; bitsPerSymbolMod input uint8; last_out output boolean; packed_data output uint8; bitsPerSymbolHeader parameter uint8; data input uint8; payload input boolean; rst input boolean; valid output boolean; counter local; decoding output boolean; err output boolean
